simulink model "EV_thermal_charger_2015a_20200311"  (R2015a)
settings: Solver=ode3  StartTime=0.0  StopTime=1800  FixedStep=sampling_time  RelTol=1e-3
PreLoadFcn:
  | run('init_setting.m')
PostLoadFcn:
  | set_param(gcs, 'SimulationCommand', 'update');
  | load('save_param/save_P_Charger', 'P_Charger');
  | load('save_param/save_T_User_set_temp_degC','T_User_set_temp_degC');
  | load('save_param/save_ENV_PNT_PTTH_Temp_add_degC','ENV_PNT_PTTH_Temp_add_degC');
  | load('save_param/save_ENV_PNT_CABIN_Temp_add_degC','ENV_PNT_CABIN_Temp_add_degC');
  | load('save_param/save_ENV_PNT_PHI_Sunlight_W','ENV_PNT_PHI_Sunlight_W');
  | load('save_param/save_ENV_PNT_Outside_Temp_ini_degC','ENV_PNT_Outside_Temp_ini_degC');
undefined symbols (not defined in the file or in its folder): BK_PNT_Pow_UL, BK_PNT_ReGene_vel_limit_DN_kmph, BK_PNT_ReGene_vel_limit_UP_kmph, BK_PNT_Tau_brake, Brk_LL, Brk_PGain, Brk_UL, BT_PNT_Hi_C_pol_hi_batt, BT_PNT_Hi_Capa_hi_batt_F, BT_PNT_Hi_ocv_SOC_hi_batt_OCV_V_table, BT_PNT_Hi_ocv_SOC_hi_batt_OCV_V_table_x_SOC, BT_PNT_Hi_R_hi_batt_cell, BT_PNT_Hi_R_pol_hi_batt, BT_PNT_Hi_SOC_MAX_hi_batt, BT_PNT_Hi_SOC_MIN_hi_batt, BT_PNT_Hi_SOC_START_hi_batt, BT_PNT_Lo_Capa_lo_batt_F, BT_PNT_Lo_ocv_SOC_lo_batt_OCV_V_table, BT_PNT_Lo_ocv_SOC_lo_batt_OCV_V_table_x_SOC, BT_PNT_Lo_R_lo_batt_ohm, BT_PNT_Lo_SOC_MAX_lo_batt, BT_PNT_Lo_SOC_MIN_lo_batt, BT_PNT_Lo_SOC_START_lo_batt, BTTH_CNT_P_BT_Heater_W, BTTH_CNT_P_BT_Heater_W_x_BTCells_degC, BTTH_CNT_Voltage_BTFan_V, BTTH_CNT_Voltage_BTFan_V_x_BTCells_degC, BTTH_PNT_BT_Heat_Resi_KpW, BTTH_PNT_BT_Heat_Resi_KpW_x_Wind_m3ps, BTTH_PNT_BT_Heater2BTCells_Heat_Resi_KpW, BTTH_PNT_BT_Heater_Heat_Capa_JpK, BTTH_PNT_BTBlock2BTAir_Heat_Resi_KpW, BTTH_PNT_BTBlock_Heat_Capa_JpK, BTTH_PNT_BTCells2BTBlock_Heat_Resi_KpW, BTTH_PNT_BTCells_Heat_Capa_JpK, BTTH_PNT_v_BTFan_Wind_vel_mps, BTTH_PNT_v_BTFan_Wind_vel_mps_x_V_BTFan, CATH_CNT_P_Aircon_W_LL, CATH_CNT_P_Aircon_W_UL, CATH_CNT_P_Gain_Aircon, CATH_CNT_P_Gain_PTC_Heater, CATH_CNT_P_Gain_SeatHT, CATH_CNT_P_PTC_Heater, CATH_CNT_P_PTC_Heater_W_LL, CATH_CNT_P_PTC_Heater_W_UL, CATH_CNT_P_PTC_Heater_x_T_Outside_temp_degC, CATH_CNT_P_SeatHT_W_LL, CATH_CNT_P_SeatHT_W_UL, CATH_CNT_PGain_Temp_blowout, CATH_CNT_T_Aircon_Indoor_degC, CATH_CNT_T_Aircon_Indoor_degC_x_T_blowout_degC, CATH_CNT_T_PTC_Heater_degC_UL, CATH_CNT_T_SeatHT_Temp_degC, CATH_CNT_T_SeatHT_Temp_degC_x_T_blowout_degC, CATH_CNT_V_HVAC_Fan, CATH_CNT_V_HVAC_Fan_x_T_blowout_degC, CATH_CNT_V_RDFan_V, CATH_CNT_V_RDFan_x_P_Aircon_W, CATH_PNT_Air_Convection_Heat_Resi_KpW, CATH_PNT_Air_Convection_Heat_Resi_x_mps ... (+141)
undefined symbols (not defined in the file): ACC_D_Gain, ACC_I_Gain, ACC_P_Gain
libraries: METI_Lib_vehicle_model x52, simulink x35
(part 2 of 6)

== system EV_thermal_charger_2015a_20200311/Vehicle/BT_Lo_PNT ==
  note: SOC算出
  note: 内部抵抗
  note: OCV電圧算出
  I_BT_Lo_PNT_A : Inport
  Cal_SOC : Subsystem
  Capa_batt(Ah) : Constant  Value=BT_PNT_Lo_Capa_lo_batt_F
  Memory6 : Memory  InheritSampleTime=on
  P_cal : METI_Lib_vehicle_model/P_cal  Type_energy=電気  Type_output_energy=出力  Power_name=Po_  t_Workspace_Name=BT_PNT_Lo_ELEC  P_VariableName=Po_BT_PNT_Lo_ELEC  Across_VariableName=V_BT_PNT_Lo_ELEC  Throgh_VariableName=I_BT_PNT_Lo_ELEC
  P_cal1 : METI_Lib_vehicle_model/P_cal  Type_energy=電気  Type_output_energy=損失  Power_name=Pl_  t_Workspace_Name=BT_PNT_Lo_ELEC_LOSS  P_VariableName=Pl_BT_PNT_Lo_ELEC_LOSS  Across_VariableName=V_BT_PNT_Lo_ELEC_LOSS  Throgh_VariableName=I_BT_PNT_Lo_ELEC_LOSS
  SOC_MAX(%) : Constant  Value=BT_PNT_Lo_SOC_MAX_lo_batt
  SOC_MIN(%) : Constant  Value=BT_PNT_Lo_SOC_MIN_lo_batt
  SOC_START(%) : Constant  Value=BT_PNT_Lo_SOC_START_lo_batt
  Subsystem : Subsystem
  Sum : Sum
  Terminator1 : Terminator
  Terminator2 : Terminator
  map_OCV : Lookup  InputValues=BT_PNT_Lo_ocv_SOC_lo_batt_OCV_V_table_x_SOC  Table=BT_PNT_Lo_ocv_SOC_lo_batt_OCV_V_table  LookUpMeth=Interpolation-Use End Values
  "V_BT_Lo_PNT_V " : Outport
  tag scope: tScope_SOC_LoBatt=global
  wires:
  Capa_batt(Ah)/1 -> Cal_SOC/2(Capa_batt)
  SOC_START(%)/1 -> Cal_SOC/3(SOC_st)
  SOC_MAX(%)/1 -> Cal_SOC/4(SOC_MAX)
  SOC_MIN(%)/1 -> Cal_SOC/5(SOC_MIN)
  Sum/1 -> "V_BT_Lo_PNT_V "/1, P_cal/1  "volt_BT_PNT_Lo_V"
  map_OCV/1 -> Sum/1
  Subsystem/1(V_BT_PNT_Lo_V) -> P_cal1/1, Sum/2
  P_cal/1 -> Terminator2/1
  P_cal1/1 -> Terminator1/1
  I_BT_Lo_PNT_A/1 -> Memory6/1, P_cal/2
  Cal_SOC/1(SOC_out) -> map_OCV/1, [tScope_SOC_LoBatt]  "SOC_BT_PNT_Lo_PCT"
  Memory6/1 -> Subsystem/1(I_BT_PNT_Lo_A), P_cal1/2, Cal_SOC/1(I_Lo_BT_PNT_A)

== system EV_thermal_charger_2015a_20200311/Vehicle/CATH_CNT ==
  note: ヒートポンプパワー＞0 → 車室への熱量＞0 ＝暖房
      |
      | ヒートポンプ パワー＜0 → 車室への熱量＜0 ＝冷房
  tSetting_P_Charger : Inport
  tSetting_T_User_set_temp_degC : Inport  Port=2
  T_ATM_PNT_Outside_degC : Inport  Port=3
  T_CABA_PNT_degC : Inport  Port=4
  T_SH_PNT_degC : Inport  Port=5
  T_AC_PNT_Indoor_degC : Inport  Port=6
  T_PTC_PNT_degC : Inport  Port=7
  v_vehicle_mps_1 : Inport  Port=8
  Calc_Temp_Blowout : Subsystem
  P_Heatpomp_Power_tgt_calc : Subsystem
  P_PTC_Heater_tgt_calc : Subsystem
  Subsystem1 : Subsystem
  T_SeatHT_Temp_tgt_calc : Subsystem
  Terminator1 : Terminator
  V_HVAC_Fan_calc : Subsystem
  V_CATH_CNT_Aircon_Fan_V : Outport
  P_CATH_CNT_Heatpomp_W : Outport  Port=2
  req_V_CATH_CNT_RDFan_V : Outport  Port=3
  P_CATH_CNT_PTC_Heater_W : Outport  Port=4
  P_CATH_CNT_SeatHT_W : Outport  Port=5
  wires:
  tSetting_T_User_set_temp_degC/1 -> Calc_Temp_Blowout/1(tSetting_T_User_set_temp_degC)  "tSetting_T_User_set_temp_degC"
  T_ATM_PNT_Outside_degC/1 -> P_PTC_Heater_tgt_calc/1(T_ATM_PNT_Outside_degC), Calc_Temp_Blowout/2(T_ATM_PNT_Outside_degC)  "T_ATM_PNT_Outside_degC"
  T_CABA_PNT_degC/1 -> Calc_Temp_Blowout/3(T_CABA_PNT_T)  "T_CABA_PNT_T"
  Calc_Temp_Blowout/2(T_diff_temp_degC) -> T_SeatHT_Temp_tgt_calc/1(T_diff_temp_degC), P_Heatpomp_Power_tgt_calc/1(T_diff_temp_degC), V_HVAC_Fan_calc/1(T_diff_temp_degC)  "制御用温度差分"
  T_SH_PNT_degC/1 -> T_SeatHT_Temp_tgt_calc/2(T_SH_PNT_degC)  "T_SH_PNT_degC"
  T_AC_PNT_Indoor_degC/1 -> P_Heatpomp_Power_tgt_calc/2(T_AC_PNT_Indoor_degC)  "T_AC_PNT_Indoor_degC"
  T_PTC_PNT_degC/1 -> P_PTC_Heater_tgt_calc/2(T_PTC_PNT_degC)  "T_PTC_PNT_degC"
  V_HVAC_Fan_calc/1(V_CATH_CNT_Aircon_Fan_V) -> V_CATH_CNT_Aircon_Fan_V/1
  P_Heatpomp_Power_tgt_calc/1(P_CATH_CNT_Heatpomp_W) -> P_CATH_CNT_Heatpomp_W/1
  P_PTC_Heater_tgt_calc/1(P_CATH_CNT_PTC_Heater_W) -> P_CATH_CNT_PTC_Heater_W/1
  T_SeatHT_Temp_tgt_calc/1(P_CATH_CNT_SeatHT_W) -> P_CATH_CNT_SeatHT_W/1
  P_Heatpomp_Power_tgt_calc/2(req_V_CATH_CNT_RDFan_V) -> req_V_CATH_CNT_RDFan_V/1
  Calc_Temp_Blowout/1(T_blowout_degC) -> Terminator1/1
  v_vehicle_mps_1/1 -> Calc_Temp_Blowout/4(v_vehicle_mps_1)  "v_vehicle_mps_1"
  Subsystem1/2(Flag_AutoWind) -> P_PTC_Heater_tgt_calc/4(Flag_AutoWind), P_Heatpomp_Power_tgt_calc/4(Flag_AutoWind), V_HVAC_Fan_calc/2(Flag_AutoWind_ON)
  Subsystem1/1(Flag_Aircon) -> P_PTC_Heater_tgt_calc/3(Flag_Aircon), P_Heatpomp_Power_tgt_calc/3(Flag_Aircon)
  tSetting_P_Charger/1 -> Subsystem1/1(tSetting_P_Charger)  "tSetting_P_Charger"

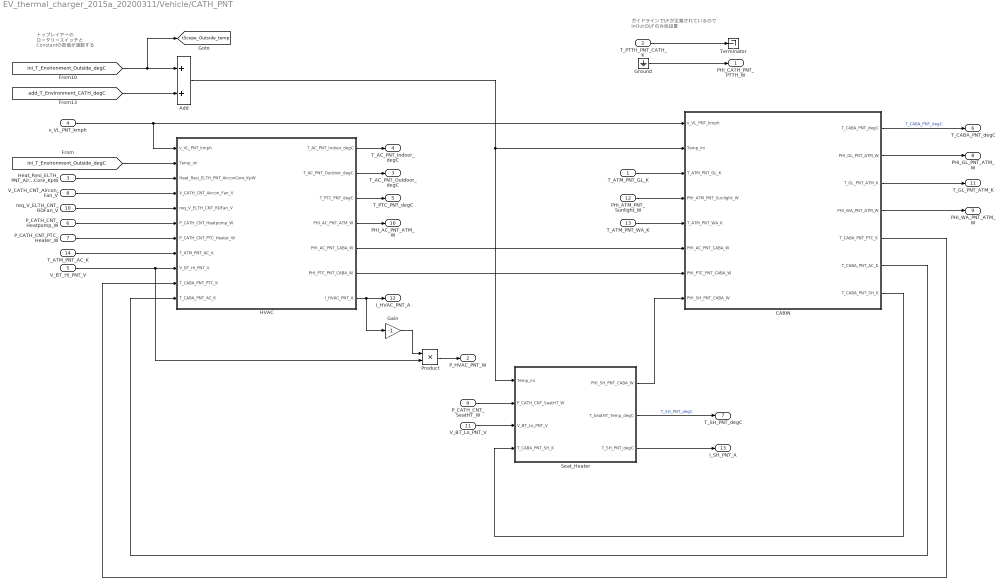
== system EV_thermal_charger_2015a_20200311/Vehicle/CATH_PNT ==
  note: トップレイヤーの
      | ロータリースイッチと
      | Constantの数値が連動する
  note: ガイドラインでI/Fが定義されているので
      | InOutのI/Fのみ仮設置
  T_ATM_PNT_GL_K : Inport
  T_PTTH_PNT_CATH_K : Inport  Port=2
  Heat_Resi_ELTH_PNT_AirconCore_KpW : Inport  Port=3
  v_VL_PNT_kmph : Inport  Port=4
  V_BT_Hi_PNT_V : Inport  Port=5
  P_CATH_CNT_Heatpomp_W : Inport  Port=6
  P_CATH_CNT_PTC_Heater_W : Inport  Port=7
  V_CATH_CNT_Aircon_Fan_V : Inport  Port=8
  P_CATH_CNT_SeatHT_W : Inport  Port=9
  req_V_ELTH_CNT_RDFan_V : Inport  Port=10
  V_BT_Lo_PNT_V : Inport  Port=11
  PHI_ATM_PNT_Sunlight_W : Inport  Port=12
  T_ATM_PNT_WA_K : Inport  Port=13
  T_ATM_PNT_AC_K : Inport  Port=14
  Add : Sum
  CABIN : Subsystem
      mask Display: image(imread('自動車　EV車両.jpg'))
  Gain : Gain  Gain=-1
  Ground : Ground
  HVAC : Subsystem
      mask Display: image(imread('熱マネ　カーエアコン.jpg'))
  Product : Product
  Seat_Heater : Subsystem
  Terminator : Terminator
  PHI_CATH_PNT_PTTH_W : Outport
  P_HVAC_PNT_W : Outport  Port=2
  T_AC_PNT_Outdoor_degC : Outport  Port=3
  T_AC_PNT_Indoor_degC : Outport  Port=4
  T_PTC_PNT_degC : Outport  Port=5
  T_CABA_PNT_degC : Outport  Port=6
  T_SH_PNT_degC : Outport  Port=7
  PHI_GL_PNT_ATM_W : Outport  Port=8
  PHI_WA_PNT_ATM_W : Outport  Port=9
  PHI_AC_PNT_ATM_W : Outport  Port=10
  T_GL_PNT_ATM_K : Outport  Port=11
  I_HVAC_PNT_A : Outport  Port=12
  I_SH_PNT_A : Outport  Port=13
  tag scope: tScope_Outside_temp=global
  wires:
  HVAC/7(I_HVAC_PNT_A) -> I_HVAC_PNT_A/1, Gain/1
  Product/1 -> P_HVAC_PNT_W/1
  CABIN/6(T_CABA_PNT_AC_K) -> HVAC/11(T_CABA_PNT_AC_K)
  CABIN/5(T_CABA_PNT_PTC_K) -> HVAC/10(T_CABA_PNT_PTC_K)
  V_BT_Lo_PNT_V/1 -> Seat_Heater/3(V_BT_Lo_PNT_V)
  Seat_Heater/3(T_SH_PNT_degC) -> I_SH_PNT_A/1
  P_CATH_CNT_SeatHT_W/1 -> Seat_Heater/2(P_CATH_CNT_SeatHT_W)
  CABIN/7(T_CABA_PNT_SH_K) -> Seat_Heater/4(T_CABA_PNT_SH_K)
  T_ATM_PNT_AC_K/1 -> HVAC/8(T_ATM_PNT_AC_K)
  CABIN/1(T_CABA_PNT_degC) -> T_CABA_PNT_degC/1  "T_CABA_PNT_degC"
  CABIN/3(T_GL_PNT_ATM_K) -> T_GL_PNT_ATM_K/1
  PHI_ATM_PNT_Sunlight_W/1 -> CABIN/4(PHI_ATM_PNT_Sunlight_W)
  T_ATM_PNT_GL_K/1 -> CABIN/3(T_ATM_PNT_GL_K)
  CABIN/2(PHI_GL_PNT_ATM_W) -> PHI_GL_PNT_ATM_W/1
  T_ATM_PNT_WA_K/1 -> CABIN/5(T_ATM_PNT_WA_K)
  CABIN/4(PHI_WA_PNT_ATM_W) -> PHI_WA_PNT_ATM_W/1
  Seat_Heater/1(PHI_SH_PNT_CABA_W) -> CABIN/8(PHI_SH_PNT_CABA_W)
  HVAC/6(PHI_PTC_PNT_CABA_W) -> CABIN/7(PHI_PTC_PNT_CABA_W)
  HVAC/5(PHI_AC_PNT_CABA_W) -> CABIN/6(PHI_AC_PNT_CABA_W)
  HVAC/4(PHI_AC_PNT_ATM_W) -> PHI_AC_PNT_ATM_W/1
  v_VL_PNT_kmph/1 -> HVAC/1(v_VL_PNT_kmph), CABIN/1(v_VL_PNT_kmph)
  V_CATH_CNT_Aircon_Fan_V/1 -> HVAC/4(V_CATH_CNT_Aircon_Fan_V)
  req_V_ELTH_CNT_RDFan_V/1 -> HVAC/5(req_V_ELTH_CNT_RDFan_V)
  P_CATH_CNT_Heatpomp_W/1 -> HVAC/6(P_CATH_CNT_Heatpomp_W)
  P_CATH_CNT_PTC_Heater_W/1 -> HVAC/7(P_CATH_CNT_PTC_Heater_W)
  HVAC/1(T_AC_PNT_Indoor_degC) -> T_AC_PNT_Indoor_degC/1
  HVAC/2(T_AC_PNT_Outdoor_degC) -> T_AC_PNT_Outdoor_degC/1
  HVAC/3(T_PTC_PNT_degC) -> T_PTC_PNT_degC/1
  V_BT_Hi_PNT_V/1 -> HVAC/9(V_BT_Hi_PNT_V), Product/2
  Seat_Heater/2(T_SeatHT_Temp_degC) -> T_SH_PNT_degC/1  "T_SH_PNT_degC"
  Heat_Resi_ELTH_PNT_AirconCore_KpW/1 -> HVAC/3(Heat_Resi_ELTH_PNT_AirconCore_KpW)
  Ground/1 -> PHI_CATH_PNT_PTTH_W/1
  T_PTTH_PNT_CATH_K/1 -> Terminator/1
  [ini_T_Environment_Outside_degC] -> HVAC/2(Temp_ini)
  [add_T_Environment_CATH_degC] -> Add/2
  [ini_T_Environment_Outside_degC] -> Add/1, [tScope_Outside_temp]
  Add/1 -> Seat_Heater/1(Temp_ini), CABIN/2(Temp_ini)
  Gain/1 -> Product/1

== system EV_thermal_charger_2015a_20200311/Vehicle/CHG_CNT ==
  note: 0：接続ネゴシエーション
      | 1：初期充電
      | 2：本充電
  note: 本充電開始時間
  note: 初期充電開始時間
  note: 充電信号
      | 充電中は1(=ON)とする
  tSetting_P_Charger : Inport
  V_CHG_PNT_V : Inport  Port=2
  SOC_BT_Hi_PNT_per : Inport  Port=3
  Add : Sum
  Charge_Current_calc : Subsystem
  Compare To Zero : simulink/Logic and Bit Operations/Compare To Zero  relop=>  OutDataTypeStr=boolean
  Constant : Constant  Value=sampling_time
  Constant1 : Constant
  Constant2 : Constant  Value=sampling_time
  Constant3 : Constant  Value=3
  Constant8 : Constant  Value=CHG_CNT_charge_UL_SOC
  Current_rate_limitter : Subsystem
  counter : Subsystem
  counter1 : Subsystem
  tgt_I_CHG_CNT_Charge_A : Outport
  wires:
  tSetting_P_Charger/1 -> Compare To Zero/1  "tSetting_P_Charger"
  Constant/1 -> counter/2(time_step)
  Constant1/1 -> counter/3(count_time)
  Constant2/1 -> counter1/2(time_step)
  Constant3/1 -> counter1/3(count_time)
  counter/1(Out1) -> Add/1
  counter1/1(Out1) -> Add/2
  V_CHG_PNT_V/1 -> Charge_Current_calc/2(V_CHG_PNT_Charge_V)  "V_CHG_PNT_Charge_V"
  SOC_BT_Hi_PNT_per/1 -> Current_rate_limitter/2(SOC_BT_Hi_PNT_per), Charge_Current_calc/3(SOC_BT_Hi_PNT_per)  "SOC_BT_Hi_PNT_per"
  Constant8/1 -> Current_rate_limitter/3(SOC_UL), Charge_Current_calc/4(Maximum_Hi_Batt_SOC)
  Current_rate_limitter/1(tgt_I_CHG_CNT_Charge_A) -> tgt_I_CHG_CNT_Charge_A/1
  Charge_Current_calc/1(Current_tgt) -> Current_rate_limitter/1(Current_tgt_In1)
  Add/1 -> Charge_Current_calc/1(Charge_mode)
  Compare To Zero/1 -> counter1/1(signal), counter/1(signal)

== system EV_thermal_charger_2015a_20200311/Vehicle/CHG_PNT ==
  V_BT_Hi_PNT_V : Inport
  tgt_I_CHG_CNT_Charge_A : Inport  Port=2
  Terminator : Terminator
  I_CHG_PNT_A : Outport
  V_CHG_PNT_V : Outport  Port=2
  wires:
  V_BT_Hi_PNT_V/1 -> Terminator/1, V_CHG_PNT_V/1
  tgt_I_CHG_CNT_Charge_A/1 -> I_CHG_PNT_A/1

== system EV_thermal_charger_2015a_20200311/Vehicle/DCDC_PNT ==
  note: 降圧指令
  note: 降圧
  note: DCDC効率計算
  V_BT_Hi_PNT_V : Inport
  V_BT_Lo_PNT_V : Inport  Port=2
  Add : Sum  Inputs=+-
  Constant3 : Constant  Value=DCDC_PNT_eta_conv_lo
  Controller : Subsystem
  Divide : Product  Inputs=/*
  Divide2 : Product  Inputs=/*
  Gain : Gain  Gain=-1
  Gain2 : Gain  Gain=-1
  P_cal : METI_Lib_vehicle_model/P_cal  Type_energy=電気  Type_output_energy=出力  Power_name=Po_  t_Workspace_Name=EL_PNT_DCDC_HI  P_VariableName=Po_EL_PNT_DCDC_HI  Across_VariableName=V_EL_PNT_DCDC_HI  Throgh_VariableName=I_EL_PNT_DCDC_HI
  P_cal5 : METI_Lib_vehicle_model/P_cal  Type_energy=電気  Type_output_energy=損失  Power_name=Pl_  t_Workspace_Name=EL_PNT_DCDC_eta_LOSS  P_VariableName=Pl_EL_PNT_DCDC_eta_LOSS  Across_VariableName=V_EL_PNT_DCDC_eta_LOSS  Throgh_VariableName=I_EL_PNT_DCDC_eta_LOSS
  P_cal6 : METI_Lib_vehicle_model/P_cal  Type_energy=電気  Type_output_energy=損失  Power_name=Pl_  t_Workspace_Name=EL_PNT_DCDC_RESI_LOSS  P_VariableName=Pl_EL_PNT_DCDC_RESI_LOSS  Across_VariableName=V_EL_PNT_DCDC_RESI_LOSS  Throgh_VariableName=I_EL_PNT_DCDC_RESI_LOSS
  P_cal7 : METI_Lib_vehicle_model/P_cal  Type_energy=電気  Type_output_energy=出力  Power_name=Po_  t_Workspace_Name=EL_PNT_DCDC_LO  P_VariableName=Po_EL_PNT_DCDC_LO  Across_VariableName=V_EL_PNT_DCDC_LO  Throgh_VariableName=I_EL_PNT_DCDC_LO
  Product1 : Product  RndMeth=Zero
  Product3 : Product  RndMeth=Zero
  Terminator{1..3,5} (4 alike) : Terminator
  eta_cal1 : METI_Lib_vehicle_model/eta_cal2
  resi1 : Subsystem
  降圧目標1 : Constant  Value=DCDC_PNT_Vtgt_conv_lo
  P_DCDC_PNT_W : Outport
  I_DCDC_PNT_Hi_A : Outport  Port=2
  I_DCDC_PNT_Lo_A : Outport  Port=3
  wires:
  V_BT_Hi_PNT_V/1 -> P_cal/1, Controller/2(V), Product3/2, Divide/1
  Controller/1(Gain) -> Product3/1
  Constant3/1 -> eta_cal1/1
  P_cal7/1 -> Terminator1/1
  P_cal5/1 -> Terminator3/1
  P_cal/1 -> Terminator5/1
  Product3/1 -> Product1/1, Add/1, P_cal5/1, Divide2/1
  Add/1 -> resi1/1(In1), P_cal6/1
  V_BT_Lo_PNT_V/1 -> P_cal7/1, Add/2
  resi1/1(Out1) -> I_DCDC_PNT_Lo_A/1, P_cal7/2, Product1/2, P_cal6/2
  P_cal6/1 -> Terminator2/1
  降圧目標1/1 -> Controller/1(Target V)
  Product1/1 -> eta_cal1/2
  Divide2/1 -> P_cal5/2
  Divide/1 -> P_cal/2, Gain/1
  Gain2/1 -> Divide2/2
  eta_cal1/1 -> Gain2/1
  Gain/1 -> I_DCDC_PNT_Hi_A/1
  eta_cal1/2 -> P_DCDC_PNT_W/1, Divide/2

== system EV_thermal_charger_2015a_20200311/Vehicle/DF_PNT ==
  "ｗ_TR_PNT_radps " : Inport
  w_TM_PNT_DN_radps : Inport  Port=2
  "T_DFTH_PNT_TM_K " : Inport  Port=3
  Constant4 : Constant  Value=1 / DF_PNT_DF_gear
  DriveShaft : Subsystem
  Gain : Gain  Gain=-1
  Product4 : Product  Inputs=**  RndMeth=Zero
  Product7 : Product  Inputs=**  RndMeth=Zero
  Q_cal1 : METI_Lib_vehicle_model/P_cal  Type_energy=回転運動  Type_output_energy=出力  Power_name=Po_  t_Workspace_Name=DF_PNT_MECK  P_VariableName=Po_DF_PNT_MECK  Across_VariableName=w_DF_PNT_MECK  Throgh_VariableName=tq_DF_PNT_MECK
  Q_cal4 : METI_Lib_vehicle_model/P_cal  Type_energy=回転運動  Type_output_energy=損失  Power_name=Pl_  t_Workspace_Name=DF_PNT_MECK_LOSS  P_VariableName=Pl_DF_PNT_MECK_LOSS  Across_VariableName=w_DF_PNT_MECK_LOSS  Throgh_VariableName=tq_DF_PNT_MECK_LOSS
  Terminator1 : Terminator
  Terminator3 : Terminator
  eta_DF : Constant  Value=DF_PNT_eta_DF
  eta_cal : METI_Lib_vehicle_model/eta_cal
  Trq_DF_PNT_UP_Nm : Outport
  Trq_DF_PNT_DN_Nm : Outport  Port=2
  "PHI_DF_PNT_W " : Outport  Port=3
  wires:
  w_TM_PNT_DN_radps/1 -> Product4/2, Q_cal4/1, Q_cal1/1
  eta_DF/1 -> eta_cal/1
  eta_cal/2 -> Trq_DF_PNT_UP_Nm/1, Q_cal1/2
  eta_cal/1 -> Q_cal4/2
  Q_cal1/1 -> Terminator3/1
  Q_cal4/1 -> Gain/1
  Product7/1 -> eta_cal/2
  Constant4/1 -> Product4/1, Product7/1
  Product4/1 -> DriveShaft/1("w_DF_PNT_radps ")
  DriveShaft/1("Trq_DF_PNT_Nm ") -> Product7/2
  Gain/1 -> "PHI_DF_PNT_W "/1
  "T_DFTH_PNT_TM_K "/1 -> Terminator1/1
  DriveShaft/2(Trq_DF_PNT_DN_Nm) -> Trq_DF_PNT_DN_Nm/1
  "ｗ_TR_PNT_radps "/1 -> DriveShaft/2("w_TR_PNT_radps ")

== system EV_thermal_charger_2015a_20200311/Vehicle/ELTH_CNT ==
  T_RDTH_PNT_RDCoolant_degC : Inport
  req_V_CATH_CNT_RDFan_V : Inport  Port=2
  MinMax : MinMax  Function=max  Inputs=2
  RD_Fan_Control : Lookup_n-D  NumberOfTableDimensions=1  BreakpointsForDimension1=ELTH_CNT_V_RDFan_x_T_Coolant  Table=ELTH_CNT_V_RDFan_V  InternalRulePriority=Speed  RndMeth=Simplest  InputSameDT=on
  Waterpomp_Control : Lookup_n-D  NumberOfTableDimensions=1  BreakpointsForDimension1=ELTH_CNT_V_Water_Pump_x_T_Coolant  Table=ELTH_CNT_V_Water_Pump_V  InternalRulePriority=Speed  RndMeth=Simplest  InputSameDT=on
  req_V_ELTH_CNT_RDFan_V : Outport
  V_ELTH_CNT_WP_V : Outport  Port=2
  wires:
  Waterpomp_Control/1 -> V_ELTH_CNT_WP_V/1
  RD_Fan_Control/1 -> MinMax/2
  T_RDTH_PNT_RDCoolant_degC/1 -> Waterpomp_Control/1, RD_Fan_Control/1  "T_RDTH_PNT_RDCoolant_degC"
  req_V_CATH_CNT_RDFan_V/1 -> MinMax/1  "req_V_CATH_CNT_RDFan_V"
  MinMax/1 -> req_V_ELTH_CNT_RDFan_V/1

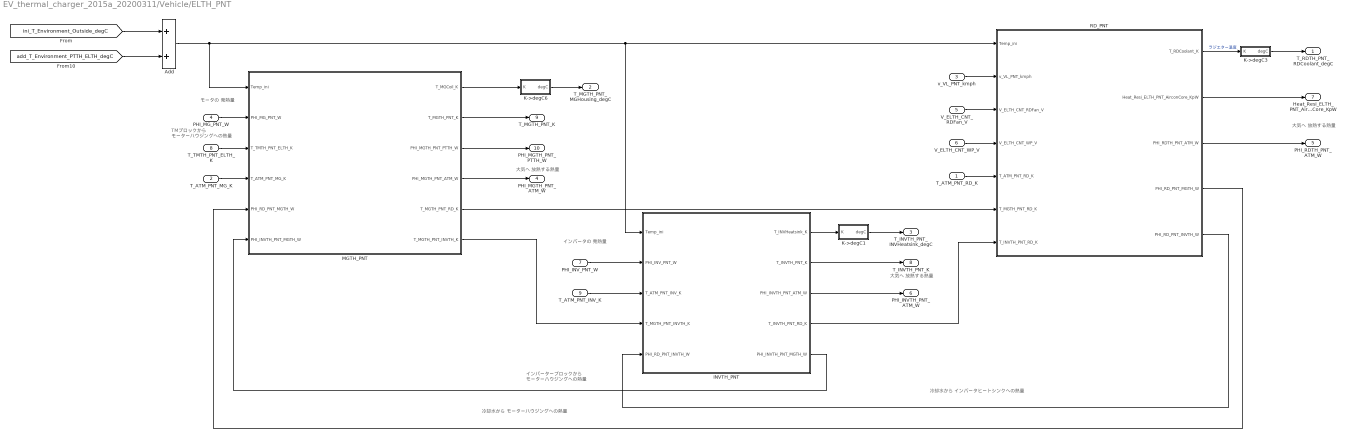
== system EV_thermal_charger_2015a_20200311/Vehicle/ELTH_PNT ==
  note: 大気へ
      | 放熱する熱量
  note: 冷却水から
      | モーターハウジングへの熱量
  note: インバーターブロックから
      | モーターハウジングへの熱量
  note: 大気へ
      | 放熱する熱量
  note: 冷却水から
      | インバータヒートシンクへの熱量
  note: モータの
      | 発熱量
  note: TMブロックから
      | モーターハウジングへの熱量
  note: インバータの
      | 発熱量
  note: 大気へ
      | 放熱する熱量
  T_ATM_PNT_RD_K : Inport
  T_ATM_PNT_MG_K : Inport  Port=2
  v_VL_PNT_kmph : Inport  Port=3
  PHI_MG_PNT_W : Inport  Port=4
  V_ELTH_CNT_RDFan_V : Inport  Port=5
  V_ELTH_CNT_WP_V : Inport  Port=6
  PHI_INV_PNT_W : Inport  Port=7
  T_TMTH_PNT_ELTH_K : Inport  Port=8
  T_ATM_PNT_INV_K : Inport  Port=9
  Add : Sum
  INVTH_PNT : Subsystem
      mask Display: image(imread('インバーター02s.jpg'))
  K->degC1 : Subsystem
  K->degC3 : Subsystem
  K->degC6 : Subsystem
  MGTH_PNT : Subsystem
      mask Display: image(imread('モータドライブシステム03.png'))
  RD_PNT : Subsystem
      mask Display: image(imread('ラジエーター_02s.jpg'))
  T_RDTH_PNT_RDCoolant_degC : Outport
  T_MGTH_PNT_MGHousing_degC : Outport  Port=2
  T_INVTH_PNT_INVHeatsink_degC : Outport  Port=3
  "PHI_MGTH_PNT_ATM_W " : Outport  Port=4
  "PHI_RDTH_PNT_ATM_W " : Outport  Port=5
  "PHI_INVTH_PNT_ATM_W " : Outport  Port=6
  Heat_Resi_ELTH_PNT_AirconCore_KpW : Outport  Port=7
  T_INVTH_PNT_K : Outport  Port=8
  T_MGTH_PNT_K : Outport  Port=9
  PHI_MGTH_PNT_PTTH_W : Outport  Port=10
  wires:
  v_VL_PNT_kmph/1 -> RD_PNT/2(v_VL_PNT_kmph)
  V_ELTH_CNT_RDFan_V/1 -> RD_PNT/3(V_ELTH_CNT_RDFan_V)
  RD_PNT/1(T_RDCoolant_K) -> K->degC3/1(K)  "ラジエター温度"
  MGTH_PNT/1(T_MGCoil_K) -> K->degC6/1(K)
  PHI_MG_PNT_W/1 -> MGTH_PNT/2(PHI_MG_PNT_W)
  MGTH_PNT/2(T_MGTH_PNT_K) -> T_MGTH_PNT_K/1
  T_TMTH_PNT_ELTH_K/1 -> MGTH_PNT/3(T_TMTH_PNT_ELTH_K)
  MGTH_PNT/3(PHI_MGTH_PNT_PTTH_W) -> PHI_MGTH_PNT_PTTH_W/1
  MGTH_PNT/6(T_MGTH_PNT_INVTH_K) -> INVTH_PNT/4(T_MGTH_PNT_INVTH_K)
  INVTH_PNT/5(PHI_INVTH_PNT_MGTH_W) -> MGTH_PNT/6(PHI_INVTH_PNT_MGTH_W)
  INVTH_PNT/2(T_INVTH_PNT_K) -> T_INVTH_PNT_K/1
  PHI_INV_PNT_W/1 -> INVTH_PNT/2(PHI_INV_PNT_W)
  INVTH_PNT/4(T_INVTH_PNT_RD_K) -> RD_PNT/7(T_INVTH_PNT_RD_K)
  RD_PNT/5(PHI_RD_PNT_INVTH_W) -> INVTH_PNT/5(PHI_RD_PNT_INVTH_W)
  MGTH_PNT/5(T_MGTH_PNT_RD_K) -> RD_PNT/6(T_MGTH_PNT_RD_K)
  RD_PNT/4(PHI_RD_PNT_MGTH_W) -> MGTH_PNT/5(" PHI_RD_PNT_MGTH_W")
  T_ATM_PNT_INV_K/1 -> INVTH_PNT/3(T_ATM_PNT_INV_K)
  INVTH_PNT/3(PHI_INVTH_PNT_ATM_W) -> "PHI_INVTH_PNT_ATM_W "/1
  T_ATM_PNT_RD_K/1 -> RD_PNT/5(T_ATM_PNT_RD_K)
  RD_PNT/3(PHI_RDTH_PNT_ATM_W) -> "PHI_RDTH_PNT_ATM_W "/1
  T_ATM_PNT_MG_K/1 -> MGTH_PNT/4(T_ATM_PNT_MG_K)
  MGTH_PNT/4(PHI_MGTH_PNT_ATM_W) -> "PHI_MGTH_PNT_ATM_W "/1
  INVTH_PNT/1(T_INVHeatsink_K) -> K->degC1/1(K)
  V_ELTH_CNT_WP_V/1 -> RD_PNT/4(V_ELTH_CNT_WP_V)
  K->degC3/1(degC) -> T_RDTH_PNT_RDCoolant_degC/1
  [add_T_Environment_PTTH_ELTH_degC] -> Add/2
  [ini_T_Environment_Outside_degC] -> Add/1
  Add/1 -> MGTH_PNT/1(Temp_ini), INVTH_PNT/1(Temp_ini), RD_PNT/1(Temp_ini)
  K->degC6/1(degC) -> T_MGTH_PNT_MGHousing_degC/1
  K->degC1/1(degC) -> T_INVTH_PNT_INVHeatsink_degC/1
  RD_PNT/2(Heat_Resi_ELTH_PNT_AirconCore_KpW) -> Heat_Resi_ELTH_PNT_AirconCore_KpW/1

== system EV_thermal_charger_2015a_20200311/Vehicle/EL_PNT ==
  note: 抵抗性負荷
  V_BT_Lo_PNT_V : Inport
  Add : Sum  Inputs=-+|
  Constant : Constant  Value=EL_PNT_R_bodyelec_lo
  Divide_0wari1 : Subsystem  mask(Divide_0割防止){}
      mask help:
      | 0割防止を行ったDivideブロックです。
      | 第2入力端子が0の場合、出力は0になります。
      mask Help:
      | 0割防止を行ったDivideブロックです。
      | 第2入力端子が0の場合、出力は0になります。
      mask Display:
      | port_label('input', 1, '×')
      | port_label('input', 2, '÷')
  Gain : Gain  Gain=-1
  Lo_body_elec_load_resi : Subsystem
  P_cal : METI_Lib_vehicle_model/P_cal  Type_energy=電気  Type_output_energy=損失  Power_name=Pl_  t_Workspace_Name=EL_PNT  P_VariableName=Pl_EL_PNT  Across_VariableName=V_EL_PNT  Throgh_VariableName=I_EL_PNT
  Terminator1 : Terminator
  V_Body_ground : Constant  Value=0
  I_EL_PNT_A : Outport
  wires:
  Divide_0wari1/1(Out1) -> Gain/1, P_cal/2
  V_BT_Lo_PNT_V/1 -> Add/2, P_cal/1
  Gain/1 -> I_EL_PNT_A/1
  P_cal/1 -> Terminator1/1
  Constant/1 -> Divide_0wari1/2(In2)
  Add/1 -> Divide_0wari1/1(In1)
  V_Body_ground/1 -> Add/1

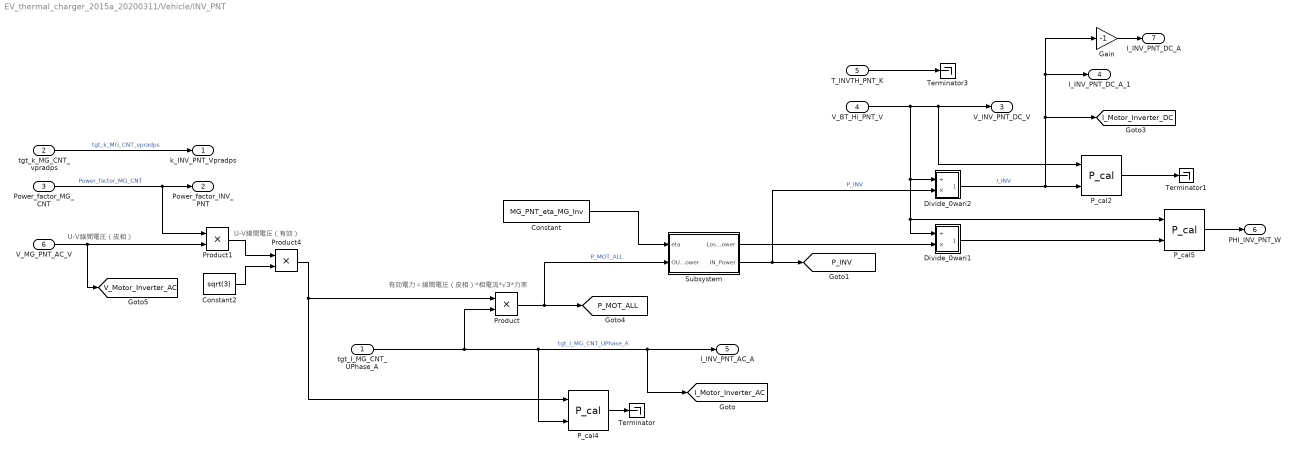
== system EV_thermal_charger_2015a_20200311/Vehicle/INV_PNT ==
  note: U-V線間電圧（皮相）
  note: 有効電力＝線間電圧（皮相）*相電流*√3*力率
  note: U-V線間電圧（有効）
  tgt_I_MG_CNT_UPhase_A : Inport
  tgt_k_MG_CNT_vpradps : Inport  Port=2
  Power_factor_MG_CNT : Inport  Port=3
  V_BT_Hi_PNT_V : Inport  Port=4
  T_INVTH_PNT_K : Inport  Port=5
  V_MG_PNT_AC_V : Inport  Port=6
  Constant : Constant  Value=MG_PNT_eta_MG_Inv
  Constant2 : Constant  Value=sqrt(3)
  Divide_0wari1 : Subsystem
  Divide_0wari2 : Subsystem
  Gain : Gain  Gain=-1
  P_cal2 : METI_Lib_vehicle_model/P_cal  Type_energy=電気  Type_output_energy=出力  Power_name=Po_  t_Workspace_Name=MG_INV_PNT_DC_ELEC  P_VariableName=Po_MG_INV_PNT_DC_ELEC  Across_VariableName=V_MG_INV_PNT_DC_ELEC  Throgh_VariableName=I_MG_INV_PNT_DC_ELEC
  P_cal4 : METI_Lib_vehicle_model/P_cal  Type_energy=電気  Type_output_energy=出力  Power_name=Po_  t_Workspace_Name=MG_INV_PNT_AC_ELEC  P_VariableName=Po_MG_INV_PNT_AC_ELEC  Across_VariableName=V_MG_INV_PNT_AC_ELEC  Throgh_VariableName=I_MG_INV_PNT_AC_ELEC
  P_cal5 : METI_Lib_vehicle_model/P_cal  Type_energy=電気  Type_output_energy=損失  Power_name=Pl_  t_Workspace_Name=MG_INV_PNT_ELEC_LOSS  P_VariableName=Pl_MG_INV_PNT_ELEC_LOSS  Across_VariableName=V_MG_INV_PNT_ELEC_LOSS  Throgh_VariableName=I_MG_INV_PNT_ELEC_LOSS
  Product : Product
  Product1 : Product
  Product4 : Product
  Subsystem : Subsystem
  Terminator : Terminator
  Terminator1 : Terminator
  Terminator3 : Terminator
  k_INV_PNT_Vpradps : Outport
  Power_factor_INV_PNT : Outport  Port=2
  V_INV_PNT_DC_V : Outport  Port=3
  I_INV_PNT_DC_A_1 : Outport  Port=4
  I_INV_PNT_AC_A : Outport  Port=5
  PHI_INV_PNT_W : Outport  Port=6
  I_INV_PNT_DC_A : Outport  Port=7
  tag scope: I_Motor_Inverter_AC=global, I_Motor_Inverter_DC=global, P_INV=global, P_MOT_ALL=global, V_Motor_Inverter_AC=global
  wires:
  Constant/1 -> Subsystem/1(eta)
  Subsystem/2(IN_Power) -> [P_INV], Divide_0wari2/2(×)  "P_INV"
  Divide_0wari1/1("　") -> P_cal5/2
  P_cal5/1 -> PHI_INV_PNT_W/1
  Subsystem/1(Loss_Power) -> Divide_0wari1/2(×)
  P_cal4/1 -> Terminator/1
  V_BT_Hi_PNT_V/1 -> P_cal2/1, V_INV_PNT_DC_V/1, Divide_0wari2/1(÷), Divide_0wari1/1(÷), P_cal5/1
  Divide_0wari2/1("　") -> [I_Motor_Inverter_DC], Gain/1, I_INV_PNT_DC_A_1/1, P_cal2/2  "I_INV"
  P_cal2/1 -> Terminator1/1
  Gain/1 -> I_INV_PNT_DC_A/1
  Product/1 -> [P_MOT_ALL], Subsystem/2(OUT_Power)  "P_MOT_ALL"
  tgt_k_MG_CNT_vpradps/1 -> k_INV_PNT_Vpradps/1  "tgt_k_MG_CNT_vpradps"
  tgt_I_MG_CNT_UPhase_A/1 -> I_INV_PNT_AC_A/1, [I_Motor_Inverter_AC], P_cal4/2, Product/2  "tgt_I_MG_CNT_UPhase_A"
  Product4/1 -> Product/1, P_cal4/1
  Power_factor_MG_CNT/1 -> Product1/1, Power_factor_INV_PNT/1  "Power_factor_MG_CNT"
  V_MG_PNT_AC_V/1 -> [V_Motor_Inverter_AC], Product1/2
  T_INVTH_PNT_K/1 -> Terminator3/1
  Constant2/1 -> Product4/2
  Product1/1 -> Product4/1

== system EV_thermal_charger_2015a_20200311/Vehicle/MG_CNT ==
  note: u相の担当トルクは
      | モータートルクの1/3
  tgt_Trq_VCU_CNT_MG_Nm : Inport
  w_MG_PNT_radps : Inport  Port=2
  V_INV_PNT_DC_V : Inport  Port=3
  Constant : Constant  Value=3
  Constant1 : Constant  Value=MG_PNT_eta_MG
  Constant2 : Constant  Value=MG_PNT_MG_Power_factor
  Divide : Product  Inputs=*/
  Divide1 : Product  Inputs=/*
  Divide2 : Product  Inputs=*/
  Memory : Memory
  Memory1 : Memory
  Memory2 : Memory
  Mux : Mux  Inputs=3
  Saturation Dynamic : simulink/Discontinuities/Saturation Dynamic  OutMin=[]  OutMax=[]  OutDataTypeStr=Inherit: Same as second input  OutDataType=fixdt(1, 16)  OutScaling=2^-10  DoSatur=off
  WeakField_Calc : Subsystem
  trq_Gurad_Calc : Subsystem
  インバータ変調率 : Constant  Value=MG_PNT_MG_mod_factor
  Power_factor_MG_CNT : Outport
  tgt_k_MG_CNT_Vpradps : Outport  Port=2
  tgt_I_MG_CNT_UPhase_A : Outport  Port=3
  tag scope: trq_MG_and_Guard=global
  wires:
  V_INV_PNT_DC_V/1 -> Memory/1  "V_INV_PNT_DC_V"
  w_MG_PNT_radps/1 -> Memory2/1  "w_MG_PNT_radps"
  trq_Gurad_Calc/2(LowerLimit) -> Mux/3, Saturation Dynamic/3
  trq_Gurad_Calc/1(UpperLimit) -> Mux/2, Saturation Dynamic/1
  Memory/1 -> WeakField_Calc/4(V_INV_PNT_DC_V)
  Saturation Dynamic/1 -> Divide/1  "U相目標トルク制限後"
  WeakField_Calc/1(k_radps2Volt_tgt) -> Divide1/1, tgt_k_MG_CNT_Vpradps/1
  Memory1/1 -> WeakField_Calc/1(I_MG_tgt)
  Divide2/1 -> Memory1/1, tgt_I_MG_CNT_UPhase_A/1
  Constant/1 -> Divide/2
  Memory2/1 -> trq_Gurad_Calc/1(w_MG_PNT_radps), WeakField_Calc/5(w_MG_PNT_radps)
  tgt_Trq_VCU_CNT_MG_Nm/1 -> Saturation Dynamic/2, Mux/1  "tgt_Trq_VCU_CNT_MG_Nm"
  Divide/1 -> Divide1/2
  Mux/1 -> [trq_MG_and_Guard]  "トルクと制限値"
  Divide1/1 -> Divide2/1
  Constant1/1 -> Divide2/2
  インバータ変調率/1 -> WeakField_Calc/3(MG_Mod_factor)
  Constant2/1 -> Power_factor_MG_CNT/1, WeakField_Calc/2(MG_Power_factor)

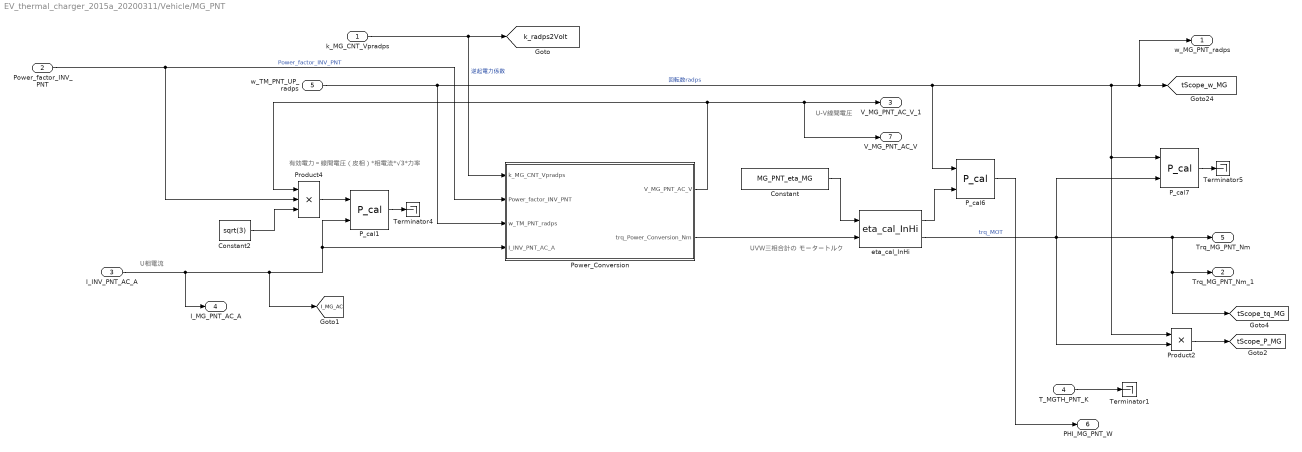
== system EV_thermal_charger_2015a_20200311/Vehicle/MG_PNT ==
  note: UVW三相合計の
      | モータートルク
  note: U-V線間電圧
  note: U相電流
  note: 有効電力＝線間電圧（皮相）*相電流*√3*力率
  k_MG_CNT_Vpradps : Inport
  Power_factor_INV_PNT : Inport  Port=2
  "I_INV_PNT_AC_A " : Inport  Port=3
  T_MGTH_PNT_K : Inport  Port=4
  w_TM_PNT_UP_radps : Inport  Port=5
  Constant : Constant  Value=MG_PNT_eta_MG
  Constant2 : Constant  Value=sqrt(3)
  P_cal1 : METI_Lib_vehicle_model/P_cal  Type_energy=電気  Type_output_energy=出力  Power_name=Po_  t_Workspace_Name=MG_PNT_ELEC  P_VariableName=Po_MG_PNT_ELEC  Across_VariableName=V_MG_PNT_ELEC  Throgh_VariableName=I_MG_PNT_ELEC
  P_cal6 : METI_Lib_vehicle_model/P_cal  Type_energy=回転運動  Type_output_energy=損失  Power_name=Pl_  t_Workspace_Name=MG_PNT_FRIC_LOSS  P_VariableName=Pl_MG_PNT_FRIC_LOSS  Across_VariableName=w_MG_PNT_FRIC_LOSS  Throgh_VariableName=tq_MG_PNT_FRIC_LOSS
  P_cal7 : METI_Lib_vehicle_model/P_cal  Type_energy=回転運動  Type_output_energy=出力  Power_name=Po_  t_Workspace_Name=MG_PNT_ROT  P_VariableName=Po_MG_PNT_ROT  Across_VariableName=w_MG_PNT_ROT  Throgh_VariableName=tq_MG_PNT_ROT
  Power_Conversion : Subsystem
  Product2 : Product
  Product4 : Product  Inputs=3
  Terminator1 : Terminator
  Terminator4 : Terminator
  Terminator5 : Terminator
  eta_cal_InHi : METI_Lib_vehicle_model/eta_cal_InHi
  w_MG_PNT_radps : Outport
  "Trq_MG_PNT_Nm_1 " : Outport  Port=2
  V_MG_PNT_AC_V_1 : Outport  Port=3
  I_MG_PNT_AC_A : Outport  Port=4
  Trq_MG_PNT_Nm : Outport  Port=5
  "PHI_MG_PNT_W " : Outport  Port=6
  "V_MG_PNT_AC_V " : Outport  Port=7
  tag scope: I_MG_AC=global, k_radps2Volt=global, tScope_P_MG=global, tScope_tq_MG=global, tScope_w_MG=global
  wires:
  P_cal1/1 -> Terminator4/1
  P_cal7/1 -> Terminator5/1
  w_TM_PNT_UP_radps/1 -> Power_Conversion/3("w_TM_PNT_radps "), w_MG_PNT_radps/1, [tScope_w_MG], Product2/1, P_cal7/1, P_cal6/1  "回転数radps"
  eta_cal_InHi/2 -> P_cal7/2, Product2/2, [tScope_tq_MG], "Trq_MG_PNT_Nm_1 "/1, Trq_MG_PNT_Nm/1  "trq_MOT"
  Product2/1 -> [tScope_P_MG]
  P_cal6/1 -> "PHI_MG_PNT_W "/1
  Constant/1 -> eta_cal_InHi/1
  eta_cal_InHi/1 -> P_cal6/2
  k_MG_CNT_Vpradps/1 -> [k_radps2Volt], Power_Conversion/1(k_MG_CNT_Vpradps)  "逆起電力係数"
  Power_Conversion/2("trq_Power_Conversion_Nm ") -> eta_cal_InHi/2
  Power_Conversion/1(V_MG_PNT_AC_V) -> Product4/1, V_MG_PNT_AC_V_1/1, "V_MG_PNT_AC_V "/1
  Product4/1 -> P_cal1/1
  "I_INV_PNT_AC_A "/1 -> [I_MG_AC], P_cal1/2, Power_Conversion/4("I_INV_PNT_AC_A "), I_MG_PNT_AC_A/1
  Power_factor_INV_PNT/1 -> Power_Conversion/2(Power_factor_INV_PNT), Product4/2  "Power_factor_INV_PNT"
  Constant2/1 -> Product4/3
  T_MGTH_PNT_K/1 -> Terminator1/1

== system EV_thermal_charger_2015a_20200311/Vehicle/PTTH_PNT ==
  note: DFブロックへ
      | 放熱する熱量
  note: DFからの熱量
  note: モーターハウジングからの熱量
  note: 大気へ
      | 放熱する熱量
  note: 大気へ
      | 放熱する熱量
  note: TMからの熱量
  note: 空調システムからの熱量
  note: ガイドラインでI/Fが定義されているので
      | InOutのI/Fのみ仮設置
  PHI_DF_PNT_W : Inport
  PHI_TM_PNT_W : Inport  Port=2
  "PHI_CATH_PNT_PTTH_W " : Inport  Port=3
  T_ATM_PNT_DF_K : Inport  Port=4
  T_ATM_PNT_TM_K : Inport  Port=5
  PHI_MGTH_PNT_PTTH_W : Inport  Port=6
  Add : Sum
  DFTH_PNT : Subsystem
      mask Display: image(imread('picture\回転変換.png'))
  Ground : Ground
  K->degC6 : Subsystem
  TMTH_PNT : Subsystem
      mask Display: image(imread('picture\image\トランスミッション02.jpg'))
  Terminator : Terminator
  T_TMTH_PNT_TM_K : Outport
  T_DFTH_PNT_TM_K : Outport  Port=2
  T_TMTH_PNT_ELTH_K : Outport  Port=3
  "PHI_DFTH_PNT_ATM_W " : Outport  Port=4
  "PHI_TMTH_PNT_ATM_W " : Outport  Port=5
  T_TMTH_PNT_TF_degC : Outport  Port=6
  T_PTTH_PNT_CATH_K : Outport  Port=7
  wires:
  TMTH_PNT/5(T_TF_K) -> K->degC6/1(K)
  DFTH_PNT/3("PHI_DFTH_PNT_TMTH_W ") -> TMTH_PNT/5("PHI_DFTH_PNT_TMTH_W ")
  TMTH_PNT/1(T_TMTH_PNT_DFTH_K) -> DFTH_PNT/4("T_TMTH_PNT_DFTH_K ")
  PHI_DF_PNT_W/1 -> DFTH_PNT/3(PHI_DF_PNT_W)
  DFTH_PNT/2(T_DFTH_PNT_TM_K) -> T_DFTH_PNT_TM_K/1
  TMTH_PNT/2(PHI_TMTH_PNT_ATM_W) -> "PHI_TMTH_PNT_ATM_W "/1
  T_ATM_PNT_TM_K/1 -> TMTH_PNT/4("T_ATM_PNT_TM_K ")
  T_ATM_PNT_DF_K/1 -> DFTH_PNT/2("T_ATM_PNT_DF_K ")
  K->degC6/1(degC) -> T_TMTH_PNT_TF_degC/1
  TMTH_PNT/4("T_TMTH_PNT_TM_K ") -> T_TMTH_PNT_TM_K/1
  PHI_TM_PNT_W/1 -> TMTH_PNT/2(PHI_TM_PNT_W)
  TMTH_PNT/3(T_TMTH_PNT_ELTH_K) -> T_TMTH_PNT_ELTH_K/1
  [add_T_Environment_PTTH_ELTH_degC] -> Add/2
  [ini_T_Environment_Outside_degC] -> Add/1
  Add/1 -> DFTH_PNT/1(Temp_ini), TMTH_PNT/1(Temp_ini)
  PHI_MGTH_PNT_PTTH_W/1 -> TMTH_PNT/3("PHI_MGTH_PNT_PTTH_W ")
  Ground/1 -> T_PTTH_PNT_CATH_K/1
  "PHI_CATH_PNT_PTTH_W "/1 -> Terminator/1
  DFTH_PNT/1("PHI_DFTH_PNT_ATM_W ") -> "PHI_DFTH_PNT_ATM_W "/1

== system EV_thermal_charger_2015a_20200311/Vehicle/TM_PNT ==
  Trq_DF_PNT_UP_Nm : Inport
  "Trq_MG_PNT_Nm " : Inport  Port=2
  T_TMTH_PNT_TM_K : Inport  Port=3
  Constant4 : Constant  Value=TM_PNT_ratio_MG2_gear
  Flywheel1 : Subsystem
  Product4 : Product  Inputs=**  RndMeth=Zero
  Product7 : Product  Inputs=**  RndMeth=Zero
  Q_cal1 : METI_Lib_vehicle_model/P_cal  Type_energy=回転運動  Type_output_energy=出力  Power_name=Po_  t_Workspace_Name=TM_PNT_MECK  P_VariableName=Po_TM_PNT_MECK  Across_VariableName=w_TM_PNT_MECK  Throgh_VariableName=tq_TM_PNT_MECK
  Q_cal4 : METI_Lib_vehicle_model/P_cal  Type_energy=回転運動  Type_output_energy=損失  Power_name=Pl_  t_Workspace_Name=TM_PNT_MECK_LOSS  P_VariableName=Pl_TM_PNT_MECK_LOSS  Across_VariableName=w_TM_PNT_MECK_LOSS  Throgh_VariableName=tq_TM_PNT_MECK_LOSS
  Terminator1 : Terminator
  Terminator2 : Terminator
  eta_DF : Constant  Value=TM_PNT_eta_MG2_gear
  eta_cal_InHi : METI_Lib_vehicle_model/eta_cal_InHi
  "w_TM_PNT_DN_radps " : Outport
  PHI_TM_PNT_W : Outport  Port=2
  w_TM_PNT_UP_radps : Outport  Port=3
  wires:
  Q_cal1/1 -> Terminator1/1
  "Trq_MG_PNT_Nm "/1 -> Q_cal1/2, eta_cal_InHi/2
  Flywheel1/1(w_TM_PNT_DN_radps) -> "w_TM_PNT_DN_radps "/1
  Trq_DF_PNT_UP_Nm/1 -> Flywheel1/1(Trq_DF_PNT_UP_Nm)
  eta_DF/1 -> eta_cal_InHi/1
  eta_cal_InHi/1 -> Q_cal4/2
  Constant4/1 -> Product7/1, Product4/1
  eta_cal_InHi/2 -> Product7/2
  Product4/1 -> Q_cal1/1, Q_cal4/1, w_TM_PNT_UP_radps/1
  Flywheel1/2("w_ROT_TM_Flywheel_UP ") -> Product4/2
  Product7/1 -> Flywheel1/2(Trq_TM_Flywheel_UP)
  Q_cal4/1 -> PHI_TM_PNT_W/1
  T_TMTH_PNT_TM_K/1 -> Terminator2/1

== system EV_thermal_charger_2015a_20200311/Vehicle/TR_PNT ==
  note: 車両を動かす側が正
  note: 車両を動かす側が正
  note: M (トルクNm) = F (力(N)） × r (タイヤ半径(m))
  note: omg (回転数rad/s) = v (車速m/s) / r (タイヤ半径(m))
  note: トルク⇔力変換
  note: 並進⇔回転変換
  note: 転がり抵抗
  "Trq_TR_PNT_Nm " : Inport
  v_VL_PNT_mps : Inport  Port=2
  Constant2 : Constant  Value=1/tire_r
  Product5 : Product  RndMeth=Zero
  Product6 : Product  RndMeth=Zero
  Sum2 : Sum  Inputs=-+|
  cal_roll_resi : METI_Lib_vehicle_model/vehicle_model/cal_roll_resi  Myu_tire=myu  Vehicle_Mass=M  Gravi_acc=g
  ｗ_TR_PNT_radps : Outport
  "F_TR_PNT_N " : Outport  Port=2
  tag scope: tScope_F_tire=global
  wires:
  "Trq_TR_PNT_Nm "/1 -> Product6/2
  Product5/1 -> ｗ_TR_PNT_radps/1  "w_TR_PNT_radps"
  v_VL_PNT_mps/1 -> Product5/1, cal_roll_resi/1
  Constant2/1 -> Product6/1, Product5/2
  Product6/1 -> Sum2/2
  cal_roll_resi/1 -> Sum2/1
  Sum2/1 -> "F_TR_PNT_N "/1, [tScope_F_tire]  "f_TR_PNT_N"

== system EV_thermal_charger_2015a_20200311/Vehicle/VCU_CNT ==
  note: 回生ブレーキ
      | 協調ブレーキ
      | あり
  note: 回生ブレーキ
      | 協調ブレーキ
      | なし
  open_break_Driver_per : Inport
  open_accel_Driver_per : Inport  Port=2
  v_VL_PNT_mps_1 : Inport  Port=3
  w_MG_PNT_radps : Inport  Port=4
  SOC_BT_Hi_PNT_per : Inport  Port=5
  P_HVAC_PNT_W : Inport  Port=6
  P_DCDC_PNT_W : Inport  Port=7
  Constant : Constant  Value=0
  Constant1 : Constant  Value=VCU_CNT_Cooperative_Control_Brake_flag
  Memory{,1..4} (5 alike) : Memory
  PDfSOC : Subsystem
  ReGenerativeBrake_Calc : Subsystem
  Switch : Switch  Criteria=u2 > Threshold
  trq_MG2_GuardCalc : Subsystem
  trq_MG2_tgtCalc2 : Subsystem
  ユーザ要求駆力算出 : Subsystem
  F_VCU_CNT_re_break_N : Outport
  tgt_Trq_VCU_CNT_MG_Nm : Outport  Port=2
  wires:
  SOC_BT_Hi_PNT_per/1 -> Memory1/1  "SOC_BT_Hi_PNT_per"
  open_accel_Driver_per/1 -> ユーザ要求駆力算出/1(open_accel_Driver_per)  "open_accel_Driver_per"
  v_VL_PNT_mps_1/1 -> Memory/1  "v_VL_PNT_mps_1"
  ユーザ要求駆力算出/1(P_vehicle_tgt) -> trq_MG2_tgtCalc2/1(User_Power_req)
  PDfSOC/2(PSoFout) -> trq_MG2_GuardCalc/3(PSoFout)
  PDfSOC/1(PSoFin) -> trq_MG2_GuardCalc/2(PSoFin)
  w_MG_PNT_radps/1 -> Memory3/1  "w_MG_PNT_radps"
  open_break_Driver_per/1 -> ユーザ要求駆力算出/2(open_break_Driver_per), ReGenerativeBrake_Calc/2(open_break_Driver_per)  "open_break_Driver_per"
  Switch/1 -> trq_MG2_tgtCalc2/6(trq_R_brake_tgt)
  P_HVAC_PNT_W/1 -> Memory4/1  "P_HVAC_PNT_W"
  ユーザ要求駆力算出/2(trq_motor_UserAcc_tgt) -> trq_MG2_tgtCalc2/3(trq_motor_UserAcc_tgt)
  trq_MG2_GuardCalc/1(trq_MG2_UpperGuard) -> trq_MG2_tgtCalc2/4(trq_MG2_UpperGuard)
  trq_MG2_GuardCalc/2(trq_MG2_LowerGuard) -> trq_MG2_tgtCalc2/5(trq_MG2_LowerGuard)
  Memory/1 -> ユーザ要求駆力算出/3(v_VL_PNT_mps_1), ReGenerativeBrake_Calc/1(v_VL_PNT_mps_1)
  Memory1/1 -> PDfSOC/1(SOC_BT_Hi_PNT_per)
  Memory3/1 -> trq_MG2_GuardCalc/1(w_MG_PNT_radps), trq_MG2_tgtCalc2/2(w_MG_PNT_radps)
  trq_MG2_tgtCalc2/2(F_VCU_CNT_re_break_N) -> F_VCU_CNT_re_break_N/1
  Memory4/1 -> trq_MG2_GuardCalc/4(P_HVAC_PNT_W)
  trq_MG2_tgtCalc2/1(tgt_Trq_VCU_CNT_MG_Nm) -> tgt_Trq_VCU_CNT_MG_Nm/1
  P_DCDC_PNT_W/1 -> Memory2/1  "P_DCDC_PNT_W"
  Memory2/1 -> trq_MG2_GuardCalc/5(P_DCDC_PNT_W)
  Constant1/1 -> Switch/2
  Constant/1 -> Switch/3
  ReGenerativeBrake_Calc/1(trq_R_brake_tgt) -> Switch/1

== system EV_thermal_charger_2015a_20200311/Vehicle/VL_PNT ==
  note: 空気抵抗
  note: 登坂抵抗
  note: 車両慣性
  F_TR_PNT_N : Inport
  P_cal : METI_Lib_vehicle_model/P_cal  Type_energy=並進運動  Type_output_energy=出力  Power_name=Po_  t_Workspace_Name=VL_PNT_TIRE_MECK  P_VariableName=Po_VL_PNT_TIRE_MECK  Across_VariableName=v_VL_PNT_TIRE_MECK  Throgh_VariableName=F_VL_PNT_TIRE_MECK
  P_cal1 : METI_Lib_vehicle_model/P_cal  Type_energy=並進運動  Type_output_energy=損失  Power_name=Pl_  t_Workspace_Name=VL_PNT_AIR_RESI  P_VariableName=Pl_VL_PNT_AIR_RESI  Across_VariableName=v_VL_PNT_AIR_RESI  Throgh_VariableName=F_VL_PNT_AIR_RESI
  P_cal3 : METI_Lib_vehicle_model/P_cal  Type_energy=並進運動  Type_output_energy=損失  Power_name=Pl_  t_Workspace_Name=VL_PNT_GRAD_RESI_MECK  P_VariableName=Pl_VL_PNT_GRAD_RESI_MECK  Across_VariableName=v_VL_PNT_GRAD_RESI_MECK  Throgh_VariableName=F_VL_PNT_GRAD_RESI_MECK
  P_cal4 : METI_Lib_vehicle_model/P_cal  Type_energy=並進運動  Type_output_energy=出力  Power_name=Po_  t_Workspace_Name=VL_PNT_VL_MASS_MECK  P_VariableName=Po_VL_PNT_VL_MASS_MECK  Across_VariableName=v_VL_PNT_VL_MASS_MECK  Throgh_VariableName=F_VL_PNT_VL_MASS_MECK
  Sum1 : Sum  Inputs=-+|
  Sum3 : Sum  Inputs=-+|
  Terminator{2..5} (4 alike) : Terminator
  V_wind : Constant  Value=0
  angle : Constant  Value=0
  cal_Air_resi : METI_Lib_vehicle_model/vehicle_model/cal_Air_resi  Vel_max=200
  cal_Hill_Climbing_Resi : Subsystem
      mask Display: image(imread('picture\登坂.JPG'))
  cal_Vehicle_Mass : METI_Lib_vehicle_model/vehicle_model/cal_Vehicle_Mass  Vehicle_Mass=M
  mps2kmph : Gain  Gain=mps2kmph
  v_VL_PNT_mps_1 : Outport
  v_VL_PNT_kmps : Outport  Port=2
  "v_VL_PNT_mps " : Outport  Port=3
  wires:
  P_cal4/1 -> Terminator2/1
  Sum1/1 -> cal_Vehicle_Mass/1, P_cal4/2
  P_cal1/1 -> Terminator5/1
  V_wind/1 -> cal_Air_resi/2
  cal_Air_resi/1 -> P_cal1/2, Sum3/1
  F_TR_PNT_N/1 -> P_cal/2, Sum3/2
  P_cal/1 -> Terminator3/1
  cal_Hill_Climbing_Resi/1(Out1) -> P_cal3/2, Sum1/1
  P_cal3/1 -> Terminator4/1
  Sum3/1 -> Sum1/2
  angle/1 -> cal_Hill_Climbing_Resi/1(In1)
  cal_Vehicle_Mass/1 -> mps2kmph/1, P_cal4/1, v_VL_PNT_mps_1/1, P_cal3/1, "v_VL_PNT_mps "/1, P_cal/1, P_cal1/1, cal_Air_resi/1  "v_VL_PNT_mps"
  mps2kmph/1 -> v_VL_PNT_kmps/1  "v_VL_PNT_kmph"

== system EV_thermal_charger_2015a_20200311/Driver/Caliculate_Opeining_Accel/FB ==
  delta_v_VL_kmph : Inport
  Acc_D_Gain : Gain  Gain=D_Gain
  Acc_I_Gain : Gain  Gain=I_Gain
  Acc_P_Gain : Gain  Gain=P_Gain
  Acc_P_Gain1 : Gain  Gain=P_Gain
  Derivative : Derivative
  Filter : Subsystem  Commented=through
  Integrator : Integrator
  Memory : Memory
  Product1 : Product
  Saturation2 : Saturate  UpperLimit=1  LowerLimit=0
  Sum : Sum  Inputs=+++
  Terminator : Terminator
  FB_open_accel_per : Outport
  wires:
  Filter/1(Out1) -> Product1/2
  Saturation2/1 -> Acc_P_Gain/1
  Acc_P_Gain/1 -> Product1/1
  Sum/1 -> FB_open_accel_per/1
  Derivative/1 -> Acc_D_Gain/1
  Integrator/1 -> Acc_I_Gain/1
  delta_v_VL_kmph/1 -> Memory/1
  Acc_I_Gain/1 -> Sum/3
  Acc_D_Gain/1 -> Sum/2
  Acc_P_Gain1/1 -> Sum/1
  Memory/1 -> Saturation2/1, Filter/1(In1), Acc_P_Gain1/1, Integrator/1, Derivative/1
  Product1/1 -> Terminator/1

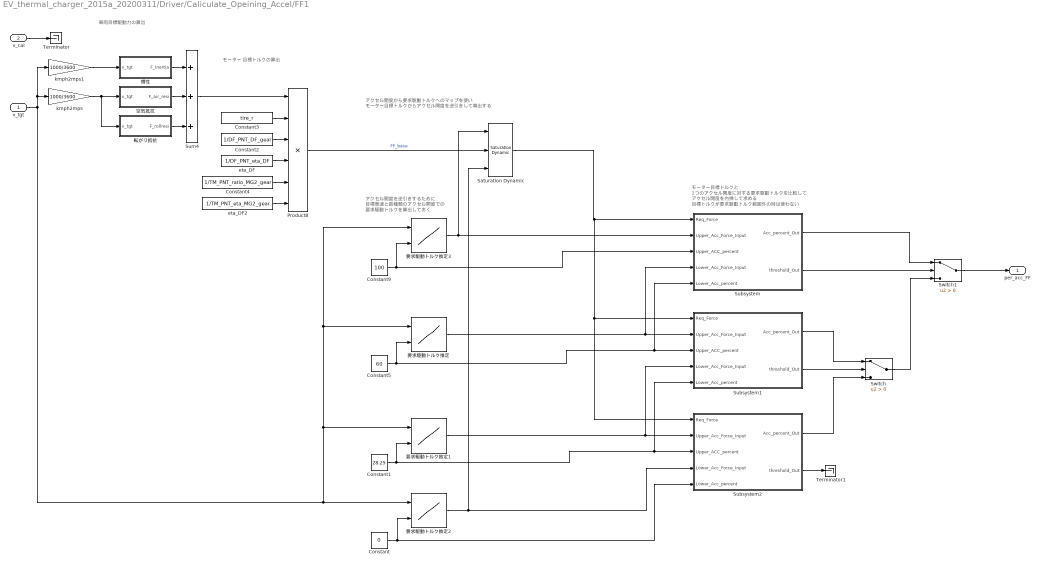
== system EV_thermal_charger_2015a_20200311/Driver/Caliculate_Opeining_Accel/FF1 ==
  note: モーター目標トルクと
      | 2つのアクセル開度に対する要求駆動トルクを比較して
      | アクセル開度を内挿して求める
      | 目標トルクが要求駆動トルク範囲外の時は使わない
  note: アクセル開度を逆引きするために
      | 目標車速と数種類のアクセル開度での
      | 要求駆動トルクを算出しておく
  note: アクセル開度から要求駆動トルクへのマップを使い
      | モーター目標トルクからアクセル開度を逆引きして導出する
  note: モーター 目標トルクの算出
  note: 車両目標駆動力の算出
  v_tgt : Inport
  v_cal : Inport  Port=2
  Constant : Constant  Value=0
  Constant1 : Constant  Value=28.25
  Constant2 : Constant  Value=1/DF_PNT_DF_gear
  Constant3 : Constant  Value=tire_r
  Constant4 : Constant  Value=1/TM_PNT_ratio_MG2_gear
  Constant5 : Constant  Value=60
  Constant9 : Constant  Value=100
  Product8 : Product  Inputs=******  RndMeth=Zero
  Saturation Dynamic : simulink/Discontinuities/Saturation Dynamic  OutMin=[]  OutMax=[]  OutDataTypeStr=Inherit: Same as second input  OutDataType=fixdt(1, 16)  OutScaling=2^-10  DoSatur=off
  Subsystem : Subsystem
  Subsystem1 : Subsystem
  Subsystem2 : Subsystem
  Sum4 : Sum  Inputs=+++
  Switch : Switch  Criteria=u2 > Threshold
  Switch1 : Switch  Criteria=u2 > Threshold
  Terminator : Terminator
  Terminator1 : Terminator
  eta_DF : Constant  Value=1/DF_PNT_eta_DF
  eta_DF2 : Constant  Value=1/TM_PNT_eta_MG2_gear
  kmph2mps : Gain  Gain=1000/3600
  kmph2mps1 : Gain  Gain=1000/3600
  慣性 : Subsystem
  空気抵抗 : Subsystem
  要求駆動トルク推定{,1..3} (4 alike) : Lookup_n-D  BreakpointsForDimension1=VCU_CNT_trq_require_v_kmph  BreakpointsForDimension2=VCU_CNT_trq_require_accper  BeginIndexSearchUsingPreviousIndexResult=on  Table=VCU_CNT_trq_require_Nm  ExtrapMethod=Clip  InternalRulePriority=Speed  RndMeth=Simplest  InputSameDT=on
  転がり抵抗 : Subsystem
  per_acc_FF : Outport
  wires:
  v_cal/1 -> Terminator/1
  kmph2mps/1 -> 空気抵抗/1(v_tgt), 転がり抵抗/1(v_tgt)
  kmph2mps1/1 -> 慣性/1(v_tgt)
  慣性/1(F_Inertia) -> Sum4/1
  転がり抵抗/1(F_rollresi) -> Sum4/3
  空気抵抗/1(F_air_resi) -> Sum4/2
  Sum4/1 -> Product8/1
  v_tgt/1 -> kmph2mps/1, kmph2mps1/1, 要求駆動トルク推定2/1, 要求駆動トルク推定1/1, 要求駆動トルク推定3/1, 要求駆動トルク推定/1
  Constant/1 -> 要求駆動トルク推定2/2, Subsystem2/5(Lower_Acc_percent)
  Constant1/1 -> 要求駆動トルク推定1/2, Subsystem2/3(Upper_ACC_percent), Subsystem1/5(Lower_Acc_percent)
  Constant5/1 -> 要求駆動トルク推定/2, Subsystem1/3(Upper_ACC_percent), Subsystem/5(Lower_Acc_percent)
  要求駆動トルク推定1/1 -> Subsystem1/4(Lower_Acc_Force_Input), Subsystem2/2(Upper_Acc_Force_Input)
  要求駆動トルク推定2/1 -> Saturation Dynamic/3, Subsystem2/4(Lower_Acc_Force_Input)
  Product8/1 -> Saturation Dynamic/2  "FF_base"
  Saturation Dynamic/1 -> Subsystem1/1(Req_Force), Subsystem2/1(Req_Force), Subsystem/1(Req_Force)
  Constant9/1 -> 要求駆動トルク推定3/2, Subsystem/3(Upper_ACC_percent)
  要求駆動トルク推定/1 -> Subsystem1/2(Upper_Acc_Force_Input), Subsystem/4(Lower_Acc_Force_Input)
  要求駆動トルク推定3/1 -> Subsystem/2(Upper_Acc_Force_Input), Saturation Dynamic/1
  Switch/1 -> Switch1/3
  Switch1/1 -> per_acc_FF/1
  Subsystem/1(Acc_percent_Out) -> Switch1/1
  Subsystem/2(threshold_Out) -> Switch1/2
  Subsystem1/2(threshold_Out) -> Switch/2
  Subsystem1/1(Acc_percent_Out) -> Switch/1
  Subsystem2/1(Acc_percent_Out) -> Switch/3
  Subsystem2/2(threshold_Out) -> Terminator1/1
  Constant3/1 -> Product8/2
  Constant2/1 -> Product8/3
  eta_DF/1 -> Product8/4
  Constant4/1 -> Product8/5
  eta_DF2/1 -> Product8/6

== system EV_thermal_charger_2015a_20200311/Driver/Caliculate_Opeining_Accel/stopmode_calc ==
  note: 停車時（＝目標車速が閾値以下の時）は
      | アクセルを踏まないようにする
  FF_FB_acc_per : Inport
  target_v_VL_kmph : Inport  Port=2
  Compare To Zero : simulink/Logic and Bit Operations/Compare To Zero  relop=>  OutDataTypeStr=boolean
  Constant2 : Constant  Value=0
  Constant6 : Constant  Value=Driver_Brake_Switch_Const2
  Subtract : Sum  Inputs=+-
  Switch : Switch  Criteria=u2 > Threshold
  open_accel_per : Outport
  wires:
  Subtract/1 -> Compare To Zero/1
  Switch/1 -> open_accel_per/1
  Compare To Zero/1 -> Switch/2
  Constant2/1 -> Switch/3
  Constant6/1 -> Subtract/2
  target_v_VL_kmph/1 -> Subtract/1
  FF_FB_acc_per/1 -> Switch/1

== system EV_thermal_charger_2015a_20200311/Vehicle/ATM_PNT/degC->K ==
  degC : Inport
  Constant2 : Constant  Value=degC2K
  Sum : Sum  Inputs=++|
  K : Outport
  wires:
  degC/1 -> Sum/2
  Constant2/1 -> Sum/1
  Sum/1 -> K/1

== system EV_thermal_charger_2015a_20200311/Vehicle/BTTH_PNT/BB_PNT ==
  note: バッテリ筐体の
      | 熱容量
  ini_T_Environment_Outside_degC : Inport
  T_ATM_PNT_BB_K : Inport  Port=2
  PHI_BTBlock1_W : Inport  Port=3
  BTBlock_Heat_Capacity : Subsystem
  BT_Block2Air_Heat_Resistance : Subsystem
  T_BTBlock1_K : Outport
  PHI_BB_PNT_ATM_W : Outport  Port=2
  T_BTBlock2_K : Outport  Port=3
  wires:
  ini_T_Environment_Outside_degC/1 -> BTBlock_Heat_Capacity/1(ini_T_Environment_Outside_degC)
  BTBlock_Heat_Capacity/1(T_BTBlock1_K) -> T_BTBlock1_K/1
  PHI_BTBlock1_W/1 -> BTBlock_Heat_Capacity/2(PHI_BTBlock1_W)
  BT_Block2Air_Heat_Resistance/1(PHI_BT2AIR_Resi1_W) -> PHI_BB_PNT_ATM_W/1
  BT_Block2Air_Heat_Resistance/2(PHI_BTBlock_Resi2_W) -> BTBlock_Heat_Capacity/3(PHI_BTBlock2_W)
  T_ATM_PNT_BB_K/1 -> BT_Block2Air_Heat_Resistance/1(T_ATM_PNT_BB_K)
  BTBlock_Heat_Capacity/2(T_BTBlock2_K) -> T_BTBlock2_K/1, BT_Block2Air_Heat_Resistance/2(T_BTBlock_Resi2_K)

== system EV_thermal_charger_2015a_20200311/Vehicle/BTTH_PNT/BC_PNT ==
  note: バッテリセルの
      | 熱容量
  PHI_BTCells4_W : Inport
  T_BTBlock_Resi1_K : Inport  Port=2
  ini_T_Environment_Outside_degC : Inport  Port=3
  PHI_BTCells2_W : Inport  Port=4
  PHI_BT_HI_PNT_W : Inport  Port=5
  BTCells_Heat_Capacity : Subsystem
  BT_Cells2BTBlock_Heat_Resistance : Subsystem
  T_BTCells4_K : Outport
  PHI_BTBlock_Resi1_W : Outport  Port=2
  T_BC_PNT_K : Outport  Port=3
  T_BTCCell_K : Outport  Port=4
  T_BTCells2_K : Outport  Port=5
  wires:
  BTCells_Heat_Capacity/2(T_BTCells2_K) -> T_BTCells2_K/1
  PHI_BTCells2_W/1 -> BTCells_Heat_Capacity/3(PHI_BTCells2_W)
  ini_T_Environment_Outside_degC/1 -> BTCells_Heat_Capacity/1(ini_T_Environment_Outside_degC)
  PHI_BT_HI_PNT_W/1 -> BTCells_Heat_Capacity/2(PHI_BTCells1_W)
  PHI_BTCells4_W/1 -> BTCells_Heat_Capacity/5(PHI_BTCells4_W)
  BT_Cells2BTBlock_Heat_Resistance/2(PHI_BTCells_Resi2_W) -> BTCells_Heat_Capacity/4(PHI_BTCells3_W)
  BT_Cells2BTBlock_Heat_Resistance/1(PHI_BTBlock_Resi1_W) -> PHI_BTBlock_Resi1_W/1
  BTCells_Heat_Capacity/1(T_BTCells1_K) -> T_BC_PNT_K/1
  T_BTBlock_Resi1_K/1 -> BT_Cells2BTBlock_Heat_Resistance/1(T_BTBlock_Resi1_K)
  BTCells_Heat_Capacity/4(T_BTCells4_K) -> T_BTCells4_K/1
  BTCells_Heat_Capacity/3(T_BTCells3_K) -> T_BTCCell_K/1, BT_Cells2BTBlock_Heat_Resistance/2(T_BTCells_Resi2_K)

== system EV_thermal_charger_2015a_20200311/Vehicle/BTTH_PNT/BF_PNT ==
  V_BTTH_CNT_BTFan_V : Inport
  T_ATM_PNT_BF_K : Inport  Port=2
  T_BT_Fan_Resi2_K : Inport  Port=3
  BTFan_Heat_Resistance : Subsystem
  BT_Fan_Heat_Resi_Calc : Subsystem
  PHI_BT_Fan_Resi2_W : Outport
  PHI_BF_PNT_ATM_W : Outport  Port=2
  wires:
  BTFan_Heat_Resistance/2(PHI_BT_Fan_Resi2_W) -> PHI_BT_Fan_Resi2_W/1
  T_BT_Fan_Resi2_K/1 -> BTFan_Heat_Resistance/3(T_BT_Fan_Resi2_K)
  T_ATM_PNT_BF_K/1 -> BTFan_Heat_Resistance/2(T_ATM_PNT_BF_K)
  BTFan_Heat_Resistance/1(PHI_BT_Fan_Resi1_W) -> PHI_BF_PNT_ATM_W/1
  V_BTTH_CNT_BTFan_V/1 -> BT_Fan_Heat_Resi_Calc/1(BTTH_PNT_Voltage_BTFan_V)
  BT_Fan_Heat_Resi_Calc/1("BTTH_PNT_BTFan_Heat_Resi_KpW ") -> BTFan_Heat_Resistance/1("BTTH_PNT_BTFan_Heat_Resi_KpW ")

== system EV_thermal_charger_2015a_20200311/Vehicle/BTTH_PNT/BH_PNT ==
  note: バッテリヒータの
      | 熱容量
  ini_T_Environment_Outside_degC : Inport
  tgt_P_BTTH_CNT_BTHeater_W : Inport  Port=2
  V_BT_Lo_PNT_V : Inport  Port=3
  T_BTCells_Resi1_K : Inport  Port=4
  BT_Heater : Subsystem
  BT_Heater2BTCells_Heat_Resistance : Subsystem
  BT_Heater_Heat_Capacity : Subsystem
  Gain : Gain  Gain=-1
  P_cal : METI_Lib_vehicle_model/P_cal  Type_energy=電気  Type_output_energy=損失  Power_name=Pl_  t_Workspace_Name=BT_Heater_Elec  P_VariableName=Pl_BT_Heater_Elec  Across_VariableName=V_BT_Heater_Elec  Throgh_VariableName=I_BT_Heater_Elec
  Terminator : Terminator
  PHI_BTCells_Resi1_W : Outport
  I_BTTH_PNT_A : Outport  Port=2
  wires:
  ini_T_Environment_Outside_degC/1 -> BT_Heater_Heat_Capacity/1(PHI_BTCells_Resi1_W)
  BT_Heater2BTCells_Heat_Resistance/1(PHI_BTCells_Resi1_W) -> PHI_BTCells_Resi1_W/1
  BT_Heater2BTCells_Heat_Resistance/2(PHI_BT_Heater_Resi2_W) -> BT_Heater_Heat_Capacity/3(PHI_BT_Heater2_W)
  BT_Heater/1(PHI_BT_Heater_W) -> BT_Heater_Heat_Capacity/2(PHI_BT_Heater1_W)
  V_BT_Lo_PNT_V/1 -> P_cal/1, BT_Heater/3(V_BT_Lo_PNT_V)
  Gain/1 -> P_cal/2
  BT_Heater/2(I_BT_Heater_A) -> I_BTTH_PNT_A/1, Gain/1
  tgt_P_BTTH_CNT_BTHeater_W/1 -> BT_Heater/2(tgt_P_BTTH_CNT_BTHeater_W)
  P_cal/1 -> Terminator/1
  BT_Heater_Heat_Capacity/1(T_BT_Heater1_K) -> BT_Heater/1(T_BT_Heater_K)
  BT_Heater_Heat_Capacity/2(T_BT_Heater2_K) -> BT_Heater2BTCells_Heat_Resistance/2(T_BT_Heater_Resi2_K)
  T_BTCells_Resi1_K/1 -> BT_Heater2BTCells_Heat_Resistance/1(T_BTCells_Resi1_K)

== system EV_thermal_charger_2015a_20200311/Vehicle/BTTH_PNT/K->degC ==
  K : Inport
  Constant2 : Constant  Value=K2degC
  Sum : Sum  Inputs=++|
  degC : Outport
  wires:
  K/1 -> Sum/2
  Constant2/1 -> Sum/1
  Sum/1 -> degC/1

== system EV_thermal_charger_2015a_20200311/Vehicle/BTTH_PNT/K->degC1 ==
  K : Inport
  Constant2 : Constant  Value=K2degC
  Sum : Sum  Inputs=++|
  degC : Outport
  wires:
  K/1 -> Sum/2
  Constant2/1 -> Sum/1
  Sum/1 -> degC/1

== system EV_thermal_charger_2015a_20200311/Vehicle/BT_Hi_PNT/Cal_SOC ==
  I_BT_PNT_A : Inport
  Capa_batt : Inport  Port=2
  SOC_st : Inport  Port=3
  SOC_MAX : Inport  Port=4
  SOC_MIN : Inport  Port=5
  Clock : Clock
  Memory : Memory
  Memory1 : Memory
  Saturation Dynamic : simulink/Discontinuities/Saturation Dynamic  OutMin=[]  OutMax=[]  OutDataTypeStr=Inherit: Same as second input  OutDataType=fixdt(1, 16)  OutScaling=2^-10  DoSatur=off
  Subsystem4 : Subsystem  mask{SOC=SOC_LoBat, VariableName=Asec_LoBat}
      mask prompts: SOC "バッテリSOC"; VariableName "バッテリ容量変化量(Asec)"
  Sum : Sum  Inputs=|++
  Sum1 : Sum  Inputs=++|
  Sum2 : Sum  Inputs=+-|
  Sum5 : Sum  Inputs=|+-
  capa_mn : Product  RndMeth=Zero
  capa_mx : Product  RndMeth=Zero
  capa_mx1 : Product  RndMeth=Zero
  capa_st : Product  RndMeth=Zero
  capa_st1 : Product  Inputs=*/  RndMeth=Zero
  h2sec : Gain  Gain=h2sec
  k : Gain  Gain=percent2mujigen
  k1 : Gain  Gain=percent2mujigen
  k2 : Gain  Gain=percent2mujigen
  k3 : Gain  Gain=mujigen2percent
  SOC_out : Outport
  wires:
  Sum5/1 -> capa_mx1/2
  Memory1/1 -> Sum5/2
  Sum/1 -> Saturation Dynamic/2
  Clock/1 -> Sum5/1, Memory1/1
  capa_mx1/1 -> Sum1/1
  k3/1 -> Subsystem4/1(In1), SOC_out/1
  Sum1/1 -> Sum/2
  Memory/1 -> Sum1/2
  k2/1 -> capa_st/2
  k1/1 -> capa_mn/2
  k/1 -> capa_mx/2
  capa_st/1 -> Sum2/2, Sum/1
  Saturation Dynamic/1 -> Sum2/1, capa_st1/1
  capa_mx/1 -> Saturation Dynamic/1
  capa_mn/1 -> Saturation Dynamic/3
  capa_st1/1 -> k3/1
  h2sec/1 -> capa_mn/1, capa_st1/2, capa_st/1, capa_mx/1
  SOC_MIN/1 -> k1/1
  SOC_MAX/1 -> k/1
  SOC_st/1 -> k2/1
  Capa_batt/1 -> h2sec/1
  I_BT_PNT_A/1 -> capa_mx1/1
  Sum2/1 -> Memory/1, Subsystem4/2(In2)
